simulink model "PiekarekLabNr4_si"  (R2022b)
settings: Solver=VariableStepAuto  StartTime=0.0  StopTime=700  RelTol=1e-3
values from neighbouring files (symbols this model uses):
  dPg = 0.2*PgN    (= 3000)    [PiekarekLabNr4.m]
  L = [k]    [PiekarekLabNr4.m]
  M = [140,1]    [PiekarekLabNr4.m]
  T0 = 20    [PiekarekLabNr4.m]
  Tp0 = (Kp*Twew0+Kd*Tzew0)/(Kp+Kd)    (= 15)    [PiekarekLabNr4.m]
settings Model: Creator=Lenovo  LastModifiedBy=Lenovo

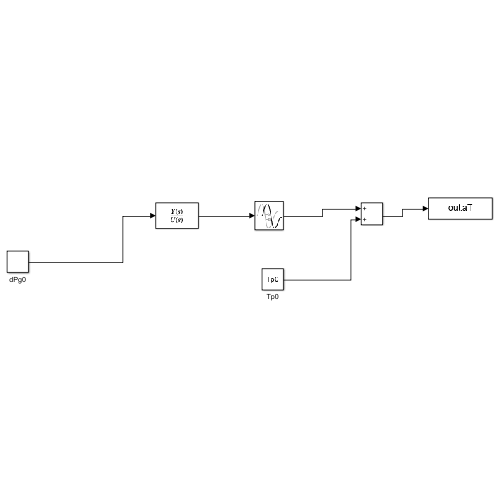
[thumbnail: Simulink's stored preview of the top-level diagram]
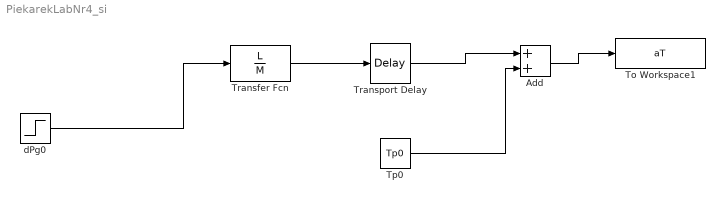
== system PiekarekLabNr4_si ==
  Add : Sum
  To Workspace1 : ToWorkspace  VariableName=aT  SampleTime=-1
  Tp0 : Constant  Value=Tp0
  Transfer Fcn : TransferFcn  Numerator=L  Denominator=M
  Transport Delay : TransportDelay  DelayTime=T0
  dPg0 : Step  Time=0  After=dPg  SampleTime=0
  wires:
  dPg0/1 -> Transfer Fcn/1
  Transfer Fcn/1 -> Transport Delay/1
  Tp0/1 -> Add/2
  Transport Delay/1 -> Add/1
  Add/1 -> To Workspace1/1
